simulink model "Fly_By_Wire_Logical_Architecture"  (R2025a)
settings: Solver=VariableStepAuto  StartTime=0.0  StopTime=10.0  RelTol=1e-3
(part 2 of 2)

== system Fly_By_Wire_Logical_Architecture/Autopilot Manager/Guidance Law ==
  Bus Element In1 : Inport  PortName=StateEstimate
  Bus Element Out1 : Outport  PortName=InitialAutocommand

== system Fly_By_Wire_Logical_Architecture/Autopilot Manager/Mode Selector ==
  Bus Element In1 : Inport  PortName=ModeCommand
  Bus Element Out1 : Outport  PortName=autoEnabled

== system Fly_By_Wire_Logical_Architecture/Flight Control Processor/Command Arbitrator ==
  Bus Element In1 : Inport  PortName=ArbitaryConfig
  Bus Element In2 : Inport  Port=2  PortName=PilotCommand
  Bus Element In3 : Inport  Port=3  PortName=AutoCommand
  Bus Element Out1 : Outport  PortName=Control Command

== system Fly_By_Wire_Logical_Architecture/Flight Control Processor/Config Manager ==
  Bus Element In1 : Inport  PortName=ConfigDemand
  Bus Element Out3 : Outport  PortName=ControlConfig
  Bus Element Out1 : Outport  Port=2  PortName=ArbitaryConfig
  Bus Element Out2 : Outport  Port=3  PortName=EstimatedConfig

== system Fly_By_Wire_Logical_Architecture/Flight Control Processor/Control Law Computer ==
  Bus Element In2 : Inport  PortName=ControlCommand
  Bus Element In1 : Inport  Port=2  PortName=ControlConfig
  Bus Element In3 : Inport  Port=3  PortName=EstimatedState
  Bus Element Out3 : Outport  PortName=CLCHealthStatusMessage
  Bus Element Out1 : Outport  Port=2  PortName=ActuatorDriveSignal
  Bus Element Out2 : Outport  Port=3  PortName=StateEstimate

== system Fly_By_Wire_Logical_Architecture/Flight Control Processor/Health Manager ==
  Bus Element In3 : Inport  PortName=CLCHealthStatusMessage
  Bus Element In2 : Inport  Port=2  PortName=SEHealthStatusMessage
  Bus Element Out1 : Outport  PortName=FCPHealthReport

== system Fly_By_Wire_Logical_Architecture/Flight Control Processor/State Estimator ==
  Bus Element In2 : Inport  PortName=ConditionedSensorData
  Bus Element In1 : Inport  Port=2  PortName=EstimatedConfig
  Bus Element Out2 : Outport  PortName=EstimatedState
  Bus Element Out1 : Outport  Port=2  PortName=SEHealthStatusMessage

== system Fly_By_Wire_Logical_Architecture/Pilot Interface Manager/CommandFormatter ==
  Bus Element In1 : Inport  PortName=FlightCommands
  Bus Element Out1 : Outport  PortName=PilotCommand

== system Fly_By_Wire_Logical_Architecture/Pilot Interface Manager/ModeSelector ==
  Bus Element In1 : Inport  PortName=FlightCommands
  Bus Element Out1 : Outport  PortName=ModeCommand

== system Fly_By_Wire_Logical_Architecture/Signal Conditioning Unit/Analog Multiplexer (MUX) ==
  Bus Element In1 : Inport  PortName=RawSensorLines
  Bus Element Out1 : Outport  PortName=SelectedSensorLines

== system Fly_By_Wire_Logical_Architecture/Signal Conditioning Unit/Analog-to-Digital Converter (ADC) ==
  Bus Element In1 : Inport  PortName=ImprovedSignal
  Bus Element Out1 : Outport  PortName=DigitalSignal

== system Fly_By_Wire_Logical_Architecture/Signal Conditioning Unit/Anti-Aliasing Noise Filter ==
  Bus Element In1 : Inport  PortName=SelectedSensorLines
  Bus Element Out2 : Outport  PortName=Health Message Report
  Bus Element Out1 : Outport  Port=2  PortName=FilteredSensorData

== system Fly_By_Wire_Logical_Architecture/Signal Conditioning Unit/Digital Filter ==
  Bus Element In1 : Inport  PortName=DigitalSignal
  Bus Element Out1 : Outport  PortName=FilteredDigitalSignal

== system Fly_By_Wire_Logical_Architecture/Signal Conditioning Unit/Digital Interface  ==
  Bus Element In1 : Inport  PortName=CorrectedSignal
  Bus Element Out1 : Outport  PortName=ConditionedSensorData

== system Fly_By_Wire_Logical_Architecture/Signal Conditioning Unit/Health Monitor ==
  Bus Element In1 : Inport  PortName=Health Message Report
  Bus Element Out1 : Outport  PortName=SCUHealthStatus

== system Fly_By_Wire_Logical_Architecture/Signal Conditioning Unit/Linearization & Calibration Logic ==
  Bus Element In1 : Inport  PortName=FilteredDigitalSignal
  Bus Element Out1 : Outport  PortName=CorrectedSignal

== system Fly_By_Wire_Logical_Architecture/Signal Conditioning Unit/Programmable Gain Amplifier (PGA) ==
  Bus Element In1 : Inport  PortName=FilteredSensorData
  Bus Element Out1 : Outport  PortName=ImprovedAnalogSignal

== system Fly_By_Wire_Logical_Architecture/Vehicle//Env Sensors/RegulationMonitor ==
  Bus Element In1 : Inport  PortName=Regulations
  Bus Element Out1 : Outport  PortName=ComplianceStatus

== system Fly_By_Wire_Logical_Architecture/Vehicle//Env Sensors/SensorSuite ==
  Bus Element In1 : Inport  PortName=PhysicalState
  Bus Element In2 : Inport  Port=2  PortName=SurfaceDeflections
  Bus Element Out1 : Outport  PortName=RawSensorLines
  Bus Element Out2 : Outport  Port=2  PortName=ActuatorFeedback

== system Fly_By_Wire_Logical_Architecture/Vehicle//Env Sensors/VehicleDynamics ==
  Bus Element In1 : Inport  PortName=ServoDriveSignal
  Bus Element In2 : Inport  Port=2  PortName=EnvironmentConditions
  Bus Element Out1 : Outport  PortName=PhysicalState
  Bus Element Out2 : Outport  Port=2  PortName=SurfaceDeflections
